simulink model "BoatBoat"  (R2020a)
settings: Solver=VariableStepAuto  StartTime=0.0  StopTime=5  RelTol=1e-3
libraries: simulink x2, fuzblock x1
settings Model: Creator=Donald  LastModifiedBy=Donald

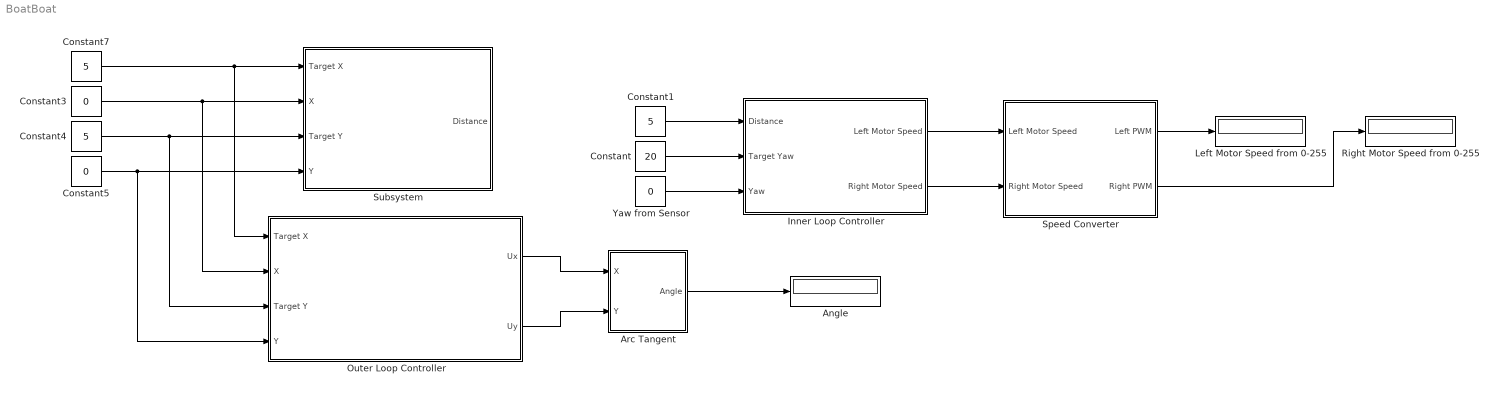
== system BoatBoat ==
  Angle : Display
  Arc Tangent : Subsystem
  Constant : Constant  Value=20
  Constant1 : Constant  Value=5
  Constant3 : Constant  Value=0
  Constant4 : Constant  Value=5
  Constant5 : Constant  Value=0
  Constant7 : Constant  Value=5
  Inner Loop Controller : Subsystem
  Left Motor Speed from 0-255 : Display
  Outer Loop Controller : Subsystem
  Right Motor Speed from 0-255 : Display
  Speed Converter : Subsystem
  Subsystem : Subsystem
  Yaw from Sensor : Constant  Value=0
  wires:
  Inner Loop Controller/1(Left Motor Speed) -> Speed Converter/1(Left Motor Speed)
  Speed Converter/1(Left PWM) -> Left Motor Speed from 0-255/1
  Speed Converter/2(Right PWM) -> Right Motor Speed from 0-255/1
  Inner Loop Controller/2(Right Motor Speed) -> Speed Converter/2(Right Motor Speed)
  Arc Tangent/1(Angle) -> Angle/1
  Yaw from Sensor/1 -> Inner Loop Controller/3(Yaw)
  Outer Loop Controller/1(Ux) -> Arc Tangent/1(X)
  Outer Loop Controller/2(Uy) -> Arc Tangent/2(Y)
  Constant7/1 -> Outer Loop Controller/1(Target X), Subsystem/1(Target X)
  Constant3/1 -> Subsystem/2(X), Outer Loop Controller/2(X)
  Constant4/1 -> Outer Loop Controller/3(Target Y), Subsystem/3(Target Y)
  Constant5/1 -> Subsystem/4(Y), Outer Loop Controller/4(Y)
  Constant/1 -> Inner Loop Controller/2(Target Yaw)
  Constant1/1 -> Inner Loop Controller/1(Distance)

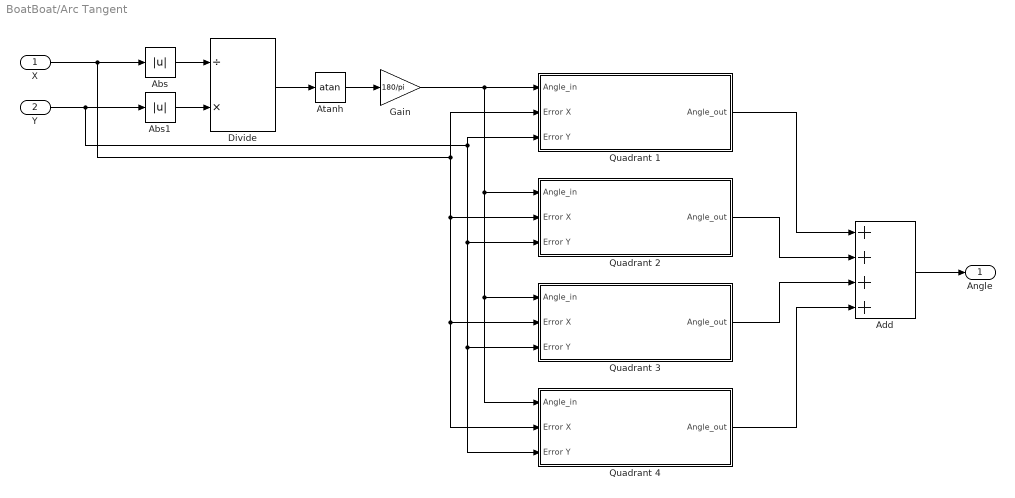
== system BoatBoat/Arc Tangent ==
  X : Inport
  Y : Inport  Port=2
  Abs : Abs
  Abs1 : Abs
  Add : Sum  Inputs=++++
  Atanh : Trigonometry  Operator=atan
  Divide : Product  Inputs=/*
  Gain : Gain  Gain=180/pi
  Quadrant 1 : Subsystem
  Quadrant 2 : Subsystem
  Quadrant 3 : Subsystem
  Quadrant 4 : Subsystem
  Angle : Outport
  wires:
  X/1 -> Quadrant 1/2(Error X), Quadrant 4/2(Error X), Quadrant 3/2(Error X), Quadrant 2/2(Error X), Abs/1
  Atanh/1 -> Gain/1
  Divide/1 -> Atanh/1
  Abs/1 -> Divide/1
  Abs1/1 -> Divide/2
  Y/1 -> Quadrant 1/3(Error Y), Quadrant 4/3(Error Y), Quadrant 3/3(Error Y), Quadrant 2/3(Error Y), Abs1/1
  Gain/1 -> Quadrant 2/1(Angle_in), Quadrant 3/1(Angle_in), Quadrant 4/1(Angle_in), Quadrant 1/1(Angle_in)
  Quadrant 1/1(Angle_out) -> Add/1
  Quadrant 2/1(Angle_out) -> Add/2
  Quadrant 3/1(Angle_out) -> Add/3
  Quadrant 4/1(Angle_out) -> Add/4
  Add/1 -> Angle/1

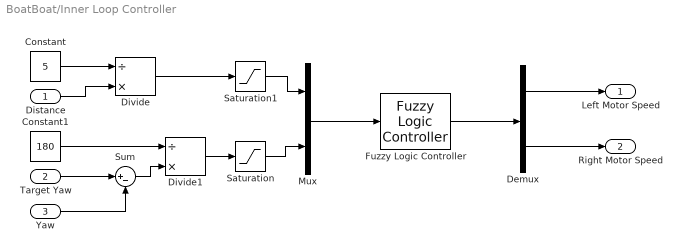
== system BoatBoat/Inner Loop Controller ==
  Distance : Inport
  Target Yaw : Inport  Port=2
  Yaw : Inport  Port=3
  Constant : Constant  Value=5
  Constant1 : Constant  Value=180
  Demux : Demux  Outputs=2
  Divide : Product  Inputs=/*
  Divide1 : Product  Inputs=/*
  Fuzzy Logic Controller : fuzblock/Fuzzy Logic  Controller  FIS='MotorMixingAlgorithm.fis'  OutputSampleNumber=101  DataType=double  FuzzifiedInputs=off  RuleFiringStrengths=off  RuleOutputs=off  AggregatedOutputs=off  SimulateUsing=Interpreted execution  OutOfRangeInputValueMessage=warning  NoRuleFiredMessage=warning  EmptyOutputFuzzySetMessage=warning
  Mux : Mux  Inputs=2
  Saturation : Saturate  UpperLimit=1  LowerLimit=-1
  Saturation1 : Saturate  UpperLimit=1  LowerLimit=0
  Sum : Sum  Inputs=|+-
  Left Motor Speed : Outport
  Right Motor Speed : Outport  Port=2
  wires:
  Fuzzy Logic Controller/1 -> Demux/1
  Mux/1 -> Fuzzy Logic Controller/1
  Target Yaw/1 -> Sum/1
  Yaw/1 -> Sum/2
  Saturation/1 -> Mux/2
  Saturation1/1 -> Mux/1
  Distance/1 -> Divide/2
  Divide/1 -> Saturation1/1
  Constant/1 -> Divide/1
  Divide1/1 -> Saturation/1
  Constant1/1 -> Divide1/1
  Sum/1 -> Divide1/2
  Demux/1 -> Left Motor Speed/1
  Demux/2 -> Right Motor Speed/1

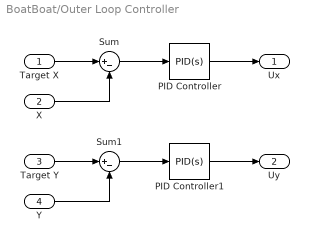
== system BoatBoat/Outer Loop Controller ==
  Target X : Inport
  X : Inport  Port=2
  Target Y : Inport  Port=3
  Y : Inport  Port=4
  PID Controller : simulink/Continuous/PID Controller  Controller=PID  Form=Parallel  TimeDomain=Continuous-time  UseExternalTs=off  SampleTime=-1  IntegratorMethod=Forward Euler  FilterMethod=Forward Euler  ControllerParametersSource=internal  P=1  I=0  D=0  UseFilter=on  N=100  TunerSelectOption=Transfer Function Based (PID Tuner App)  InitialConditionSource=internal  InitialConditionForIntegrator=0  InitialConditionForFilter=0  DifferentiatorICPrevScaledInput=0  ExternalReset=none  TrackingMode=off  Kt=1  LimitOutput=off  UpperSaturationLimit=inf  LowerSaturationLimit=-inf  LinearizeAsGain=on  AntiWindupMode=none  Kb=1  POutMin=[]  POutMax=[]  IOutMin=[]  IOutMax=[]  DOutMin=[]  DOutMax=[]  NOutMin=[]  NOutMax=[]  SumOutMin=[]  SumOutMax=[]  SaturationOutMin=[]  SaturationOutMax=[]  PParamMin=[]  PParamMax=[]  IParamMin=[]  IParamMax=[]  DParamMin=[]  DParamMax=[]  NParamMin=[]  NParamMax=[]  KbParamMin=[]  KbParamMax=[]  KtParamMin=[]  KtParamMax=[]  KbOutMin=[]  KbOutMax=[]  KtOutMin=[]  KtOutMax=[]  IntegratorOutMin=[]  IntegratorOutMax=[]  FilterOutMin=[]  FilterOutMax=[]  SumI1OutMin=[]  SumI1OutMax=[]  SumI2OutMin=[]  SumI2OutMax=[]  SumI3OutMin=[]  SumI3OutMax=[]  SumI4OutMin=[]  SumI4OutMax=[]  SumDOutMin=[]  SumDOutMax=[]  DifferentiatorOutMin=[]  DifferentiatorOutMax=[]  FilterDiffOutCoefMin=[]  FilterDiffOutCoefMax=[]  ReciprocalOutMin=[]  ReciprocalOutMax=[]  SumDenOutMin=[]  SumDenOutMax=[]  SumNumOutMin=[]  SumNumOutMax=[]  DivideOutMin=[]  DivideOutMax=[]  UdiffTsProdOutMin=[]  UdiffTsProdOutMax=[]  NTsProdOutMin=[]  NTsProdOutMax=[]  UintegralTsProdOutMin=[]  UintegralTsProdOutMax=[]  UngainTsProdOutMin=[]  UngainTsProdOutMax=[]  IntegratorContinuousStateAttributes=''  IntegratorStateMustResolveToSignalObject=off  IntegratorRTWStateStorageClass=Auto  FilterContinuousStateAttributes=''  FilterStateMustResolveToSignalObject=off  FilterRTWStateStorageClass=Auto  ParallelPVariant=InternalParameters  IdealPVariant=Disabled  IVariant=InternalParameters  DVariant=InternalParameters  IntegratorVariant=Continuous  SatVariant=Disabled  AWVariant=Passthrough  PCopyVariant=Disabled  TRVariant=Disabled  FdbkBlocksVariant=Forward  IdealPFdbkVariant=Disabled  SatFdbkVariant=Disabled  DerivativeFilterVariant=ContFilter  NVariant=InternalParameters  NCopyVariant=Disabled  FilterICVariant=InternalICsFilter  IntegratorICVariant=InternalICs  ExternalResetVariant=Disabled  TRSumVariant=Passthrough  SumFdbkVariant=Disabled  SumVariant=Sum_PID  TsampFilterVariant=InternalTs  TsampNgainVariant=Passthrough  TsampIntegralVariant=Passthrough
  PID Controller1 : simulink/Continuous/PID Controller  Controller=PID  Form=Parallel  TimeDomain=Continuous-time  UseExternalTs=off  SampleTime=-1  IntegratorMethod=Forward Euler  FilterMethod=Forward Euler  ControllerParametersSource=internal  P=1  I=0  D=0  UseFilter=on  N=100  TunerSelectOption=Transfer Function Based (PID Tuner App)  InitialConditionSource=internal  InitialConditionForIntegrator=0  InitialConditionForFilter=0  DifferentiatorICPrevScaledInput=0  ExternalReset=none  TrackingMode=off  Kt=1  LimitOutput=off  UpperSaturationLimit=inf  LowerSaturationLimit=-inf  LinearizeAsGain=on  AntiWindupMode=none  Kb=1  POutMin=[]  POutMax=[]  IOutMin=[]  IOutMax=[]  DOutMin=[]  DOutMax=[]  NOutMin=[]  NOutMax=[]  SumOutMin=[]  SumOutMax=[]  SaturationOutMin=[]  SaturationOutMax=[]  PParamMin=[]  PParamMax=[]  IParamMin=[]  IParamMax=[]  DParamMin=[]  DParamMax=[]  NParamMin=[]  NParamMax=[]  KbParamMin=[]  KbParamMax=[]  KtParamMin=[]  KtParamMax=[]  KbOutMin=[]  KbOutMax=[]  KtOutMin=[]  KtOutMax=[]  IntegratorOutMin=[]  IntegratorOutMax=[]  FilterOutMin=[]  FilterOutMax=[]  SumI1OutMin=[]  SumI1OutMax=[]  SumI2OutMin=[]  SumI2OutMax=[]  SumI3OutMin=[]  SumI3OutMax=[]  SumI4OutMin=[]  SumI4OutMax=[]  SumDOutMin=[]  SumDOutMax=[]  DifferentiatorOutMin=[]  DifferentiatorOutMax=[]  FilterDiffOutCoefMin=[]  FilterDiffOutCoefMax=[]  ReciprocalOutMin=[]  ReciprocalOutMax=[]  SumDenOutMin=[]  SumDenOutMax=[]  SumNumOutMin=[]  SumNumOutMax=[]  DivideOutMin=[]  DivideOutMax=[]  UdiffTsProdOutMin=[]  UdiffTsProdOutMax=[]  NTsProdOutMin=[]  NTsProdOutMax=[]  UintegralTsProdOutMin=[]  UintegralTsProdOutMax=[]  UngainTsProdOutMin=[]  UngainTsProdOutMax=[]  IntegratorContinuousStateAttributes=''  IntegratorStateMustResolveToSignalObject=off  IntegratorRTWStateStorageClass=Auto  FilterContinuousStateAttributes=''  FilterStateMustResolveToSignalObject=off  FilterRTWStateStorageClass=Auto  ParallelPVariant=InternalParameters  IdealPVariant=Disabled  IVariant=InternalParameters  DVariant=InternalParameters  IntegratorVariant=Continuous  SatVariant=Disabled  AWVariant=Passthrough  PCopyVariant=Disabled  TRVariant=Disabled  FdbkBlocksVariant=Forward  IdealPFdbkVariant=Disabled  SatFdbkVariant=Disabled  DerivativeFilterVariant=ContFilter  NVariant=InternalParameters  NCopyVariant=Disabled  FilterICVariant=InternalICsFilter  IntegratorICVariant=InternalICs  ExternalResetVariant=Disabled  TRSumVariant=Passthrough  SumFdbkVariant=Disabled  SumVariant=Sum_PID  TsampFilterVariant=InternalTs  TsampNgainVariant=Passthrough  TsampIntegralVariant=Passthrough
  Sum : Sum  Inputs=|+-
  Sum1 : Sum  Inputs=|+-
  Ux : Outport
  Uy : Outport  Port=2
  wires:
  X/1 -> Sum/2
  Target X/1 -> Sum/1
  Sum/1 -> PID Controller/1
  PID Controller/1 -> Ux/1
  PID Controller1/1 -> Uy/1
  Sum1/1 -> PID Controller1/1
  Target Y/1 -> Sum1/1
  Y/1 -> Sum1/2

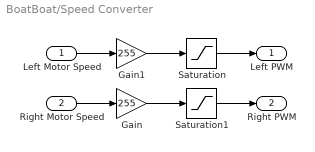
== system BoatBoat/Speed Converter ==
  Left Motor Speed : Inport
  Right Motor Speed : Inport  Port=2
  Gain : Gain  Gain=255
  Gain1 : Gain  Gain=255
  Saturation : Saturate  UpperLimit=255  LowerLimit=0
  Saturation1 : Saturate  UpperLimit=255  LowerLimit=0
  Left PWM : Outport
  Right PWM : Outport  Port=2
  wires:
  Right Motor Speed/1 -> Gain/1
  Left Motor Speed/1 -> Gain1/1
  Gain/1 -> Saturation1/1
  Gain1/1 -> Saturation/1
  Saturation/1 -> Left PWM/1
  Saturation1/1 -> Right PWM/1

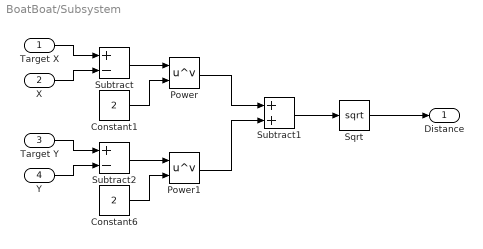
== system BoatBoat/Subsystem ==
  Target X : Inport
  X : Inport  Port=2
  Target Y : Inport  Port=3
  Y : Inport  Port=4
  Constant1 : Constant  Value=2
  Constant6 : Constant  Value=2
  Power : Math  Operator=pow  SaturateOnIntegerOverflow=on
  Power1 : Math  Operator=pow  SaturateOnIntegerOverflow=on
  Sqrt : Sqrt  SaturateOnIntegerOverflow=on
  Subtract : Sum  Inputs=+-
  Subtract1 : Sum
  Subtract2 : Sum  Inputs=+-
  Distance : Outport
  wires:
  Target Y/1 -> Subtract2/1
  Subtract/1 -> Power/1
  Power1/1 -> Subtract1/2
  Subtract2/1 -> Power1/1
  Constant6/1 -> Power1/2
  Constant1/1 -> Power/2
  Y/1 -> Subtract2/2
  Subtract1/1 -> Sqrt/1
  Power/1 -> Subtract1/1
  Sqrt/1 -> Distance/1
  Target X/1 -> Subtract/1
  X/1 -> Subtract/2

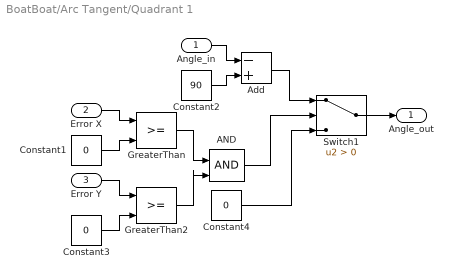
== system BoatBoat/Arc Tangent/Quadrant 1 ==
  Angle_in : Inport
  Error X : Inport  Port=2
  Error Y : Inport  Port=3
  AND : Logic  IconShape=distinctive  AllPortsSameDT=off  OutDataTypeStr=boolean
  Add : Sum  Inputs=-+
  Constant1 : Constant  Value=0
  Constant2 : Constant  Value=90
  Constant3 : Constant  Value=0
  Constant4 : Constant  Value=0
  GreaterThan : RelationalOperator  OutDataTypeStr=boolean  RndMeth=Simplest
  GreaterThan2 : RelationalOperator  OutDataTypeStr=boolean  RndMeth=Simplest
  Switch1 : Switch  Criteria=u2 > Threshold
  Angle_out : Outport
  wires:
  GreaterThan2/1 -> AND/2
  Switch1/1 -> Angle_out/1
  Constant3/1 -> GreaterThan2/2
  Error X/1 -> GreaterThan/1
  GreaterThan/1 -> AND/1
  Constant1/1 -> GreaterThan/2
  Constant4/1 -> Switch1/3
  AND/1 -> Switch1/2
  Error Y/1 -> GreaterThan2/1
  Add/1 -> Switch1/1
  Constant2/1 -> Add/2
  Angle_in/1 -> Add/1

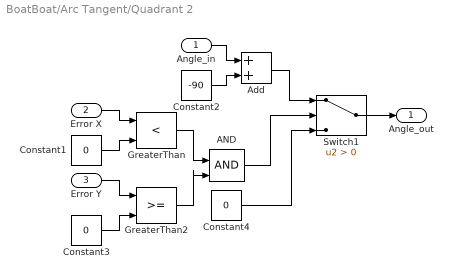
== system BoatBoat/Arc Tangent/Quadrant 2 ==
  Angle_in : Inport
  Error X : Inport  Port=2
  Error Y : Inport  Port=3
  AND : Logic  IconShape=distinctive  AllPortsSameDT=off  OutDataTypeStr=boolean
  Add : Sum
  Constant1 : Constant  Value=0
  Constant2 : Constant  Value=-90
  Constant3 : Constant  Value=0
  Constant4 : Constant  Value=0
  GreaterThan : RelationalOperator  Operator=<  OutDataTypeStr=boolean  RndMeth=Simplest
  GreaterThan2 : RelationalOperator  OutDataTypeStr=boolean  RndMeth=Simplest
  Switch1 : Switch  Criteria=u2 > Threshold
  Angle_out : Outport
  wires:
  GreaterThan2/1 -> AND/2
  Switch1/1 -> Angle_out/1
  Constant3/1 -> GreaterThan2/2
  Error X/1 -> GreaterThan/1
  GreaterThan/1 -> AND/1
  Constant1/1 -> GreaterThan/2
  Constant4/1 -> Switch1/3
  AND/1 -> Switch1/2
  Error Y/1 -> GreaterThan2/1
  Add/1 -> Switch1/1
  Constant2/1 -> Add/2
  Angle_in/1 -> Add/1

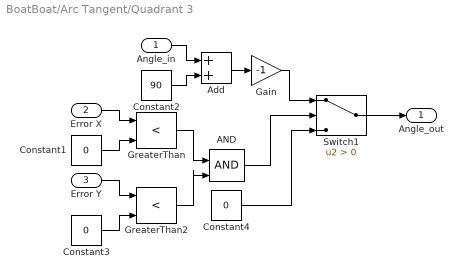
== system BoatBoat/Arc Tangent/Quadrant 3 ==
  Angle_in : Inport
  Error X : Inport  Port=2
  Error Y : Inport  Port=3
  AND : Logic  IconShape=distinctive  AllPortsSameDT=off  OutDataTypeStr=boolean
  Add : Sum
  Constant1 : Constant  Value=0
  Constant2 : Constant  Value=90
  Constant3 : Constant  Value=0
  Constant4 : Constant  Value=0
  Gain : Gain  Gain=-1
  GreaterThan : RelationalOperator  Operator=<  OutDataTypeStr=boolean  RndMeth=Simplest
  GreaterThan2 : RelationalOperator  Operator=<  OutDataTypeStr=boolean  RndMeth=Simplest
  Switch1 : Switch  Criteria=u2 > Threshold
  Angle_out : Outport
  wires:
  Angle_in/1 -> Add/1
  Constant2/1 -> Add/2
  Add/1 -> Gain/1
  Error Y/1 -> GreaterThan2/1
  AND/1 -> Switch1/2
  Constant4/1 -> Switch1/3
  Constant1/1 -> GreaterThan/2
  GreaterThan/1 -> AND/1
  Error X/1 -> GreaterThan/1
  Constant3/1 -> GreaterThan2/2
  Switch1/1 -> Angle_out/1
  GreaterThan2/1 -> AND/2
  Gain/1 -> Switch1/1

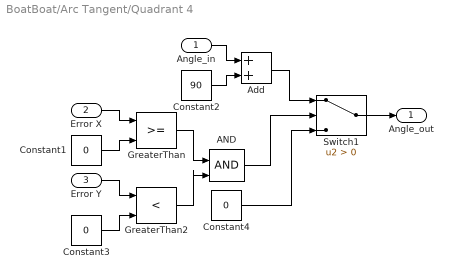
== system BoatBoat/Arc Tangent/Quadrant 4 ==
  Angle_in : Inport
  Error X : Inport  Port=2
  Error Y : Inport  Port=3
  AND : Logic  IconShape=distinctive  AllPortsSameDT=off  OutDataTypeStr=boolean
  Add : Sum
  Constant1 : Constant  Value=0
  Constant2 : Constant  Value=90
  Constant3 : Constant  Value=0
  Constant4 : Constant  Value=0
  GreaterThan : RelationalOperator  OutDataTypeStr=boolean  RndMeth=Simplest
  GreaterThan2 : RelationalOperator  Operator=<  OutDataTypeStr=boolean  RndMeth=Simplest
  Switch1 : Switch  Criteria=u2 > Threshold
  Angle_out : Outport
  wires:
  Angle_in/1 -> Add/1
  Constant2/1 -> Add/2
  Add/1 -> Switch1/1
  Error Y/1 -> GreaterThan2/1
  AND/1 -> Switch1/2
  Constant4/1 -> Switch1/3
  Constant1/1 -> GreaterThan/2
  GreaterThan/1 -> AND/1
  Error X/1 -> GreaterThan/1
  Constant3/1 -> GreaterThan2/2
  Switch1/1 -> Angle_out/1
  GreaterThan2/1 -> AND/2
